simulink model "DYC_autosar"  (R2019b)
settings: Solver=VariableStepAuto  StartTime=0.0  StopTime=10.0  RelTol=1e-3
values from neighbouring files (symbols this model uses):
  Caf = 460.0    [VehCtrlMdelDictionary.sldd]
  Car = 440.0    [VehCtrlMdelDictionary.sldd]
  dwf = 1.2    [VehCtrlMdelDictionary.sldd]
  Iz = 105.0    [VehCtrlMdelDictionary.sldd]
  Ki = 1.0    [VehCtrlMdelDictionary.sldd]
  Kp = 2.0    [VehCtrlMdelDictionary.sldd]
  lf = 0.761    [VehCtrlMdelDictionary.sldd]
  lr = 0.831    [VehCtrlMdelDictionary.sldd]
  m = 340.0    [VehCtrlMdelDictionary.sldd]
  Rt = 0.2    [VehCtrlMdelDictionary.sldd]
libraries: simulink x4
settings Model: Creator=12045  LastModifiedBy=12045
settings OptimizationCC: DefaultParameterBehavior=Inlined  EnhancedBackFolding=on  PassReuseOutputArgsAs=Individual arguments  ZeroExternalMemoryAtStartup=off  ZeroInternalMemoryAtStartup=off  OptimizeBlockOrder=speed  DifferentSizesBufferReuse=on  OptimizationCustomize=off  EfficientTunableParamExpr=on
settings DebuggingCC: ParameterTunabilityLossMsg=error
settings SFSimCC: MATLABDynamicMemAlloc=off
settings RTWCC: Description=AUTOSAR  SystemTargetFile=autosar.tlc  GenCodeOnly=on  TemplateMakefile=ert_default_tmf  GenerateReport=on  IncludeHyperlinkInReport=on  LaunchReport=on  GenerateTraceInfo=on  GenerateTraceReport=on  GenerateTraceReportSl=on  GenerateTraceReportSf=on  GenerateTraceReportEml=on
settings CodeAppCC: ForceParamTrailComments=on  IgnoreCustomStorageClasses=off  OperatorAnnotations=on  SimulinkDataObjDesc=on  SFDataObjDesc=on  InsertBlockDesc=on
settings STFCustomTargetCC: TargetLangStandard=C99 (ISO)  MultiwordLength=256  ParMdlRefBuildCompliant=on  CompOptLevelCompliant=on  IncludeMdlTerminateFcn=off  CombineOutputUpdateFcns=on  SuppressErrorStatus=on  ERTCustomFileBanners=on  SupportNonFinite=off  SupportComplex=off  SupportContinuousTime=off  SupportNonInlinedSFcns=off  RemoveResetFunc=on  MATLABClassNameForMDSCustomization=Simulink.SoftwareTarget.ERTCustomization  AutosarCompliant=on  UseToolchainInfoCompliant=on  LookupTableObjectStructAxisOrder=2,1,3,4,...  LUTObjectStructOrderEvenSpacing=Size,Table,Breakpoints  SystemTargetFile=autosar.tlc
settings ERTTargetCC: TargetLangStandard=C99 (ISO)  ConcurrentExecutionCompliant=off  IncludeMdlTerminateFcn=off  SuppressErrorStatus=on  SupportNonFinite=off  SupportComplex=off  ModelStepFunctionPrototypeControlCompliant=off  CPPClassGenCompliant=off  AutosarCompliant=on  LookupTableObjectStructAxisOrder=2,1,3,4,...  LUTObjectStructOrderEvenSpacing=Size,Table,Breakpoints  InlinedParameterPlacement=NonHierarchical  ERTCustomFileTemplate=example_file_process.tlc

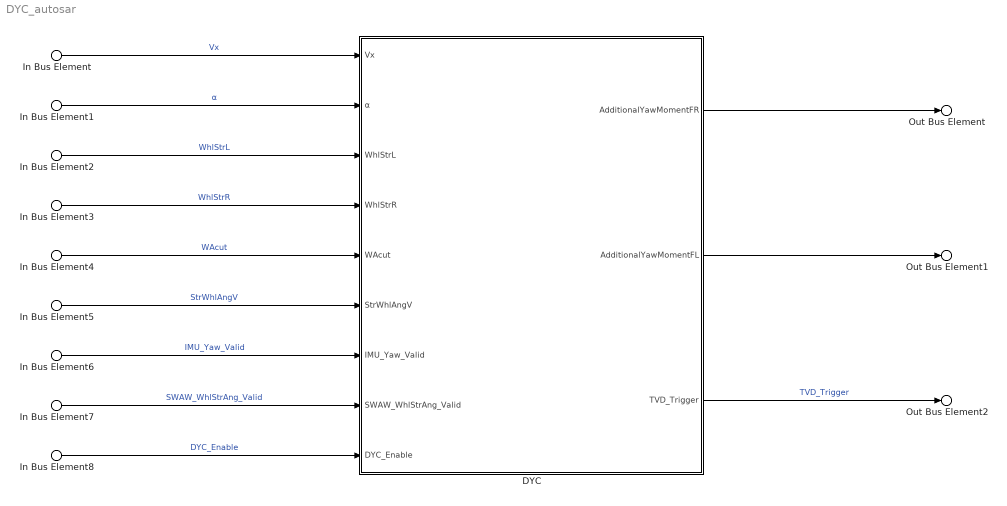
== system DYC_autosar ==
  In Bus Element : Inport  PortName=Vx  Element=Vx
  In Bus Element1 : Inport  Port=2  PortName=x0x03B1  Element=x0x03B1
  In Bus Element2 : Inport  Port=3  PortName=WhlStrL  Element=WhlStrL
  In Bus Element3 : Inport  Port=4  PortName=WhlStrR  Element=WhlStrR
  In Bus Element4 : Inport  Port=5  PortName=WAcut  Element=WAcut
  In Bus Element5 : Inport  Port=6  PortName=StrWhlAngV  Element=StrWhlAngV
  In Bus Element6 : Inport  Port=7  PortName=IMU_Yaw_Valid  Element=IMU_Yaw_Valid
  In Bus Element7 : Inport  Port=8  PortName=SWAW_WhlStrAng_Valid  Element=SWAW_WhlStrAng_Valid
  In Bus Element8 : Inport  Port=9  PortName=DYC_Enable  Element=DYC_Enable
  DYC : Subsystem
  Out Bus Element : Outport  PortName=TrqR_cmd  Element=TrqR_cmd
  Out Bus Element1 : Outport  Port=2  PortName=TrqR_cmd1  Element=TrqR_cmd1
  Out Bus Element2 : Outport  Port=3  PortName=TVD_Trigger  Element=TVD_Trigger
  wires:
  In Bus Element/1 -> DYC/1(Vx)  "Vx"
  In Bus Element1/1 -> DYC/2(α)  "α"
  In Bus Element2/1 -> DYC/3(WhlStrL)  "WhlStrL"
  In Bus Element3/1 -> DYC/4(WhlStrR)  "WhlStrR"
  In Bus Element4/1 -> DYC/5(WAcut)  "WAcut"
  In Bus Element5/1 -> DYC/6(StrWhlAngV)  "StrWhlAngV"
  In Bus Element6/1 -> DYC/7(IMU_Yaw_Valid)  "IMU_Yaw_Valid"
  In Bus Element7/1 -> DYC/8(SWAW_WhlStrAng_Valid)  "SWAW_WhlStrAng_Valid"
  In Bus Element8/1 -> DYC/9("DYC_Enable ")  "DYC_Enable"
  DYC/1(AdditionalYawMomentFR) -> Out Bus Element/1
  DYC/2(AdditionalYawMomentFL) -> Out Bus Element1/1
  DYC/3(TVD_Trigger) -> Out Bus Element2/1  "TVD_Trigger"

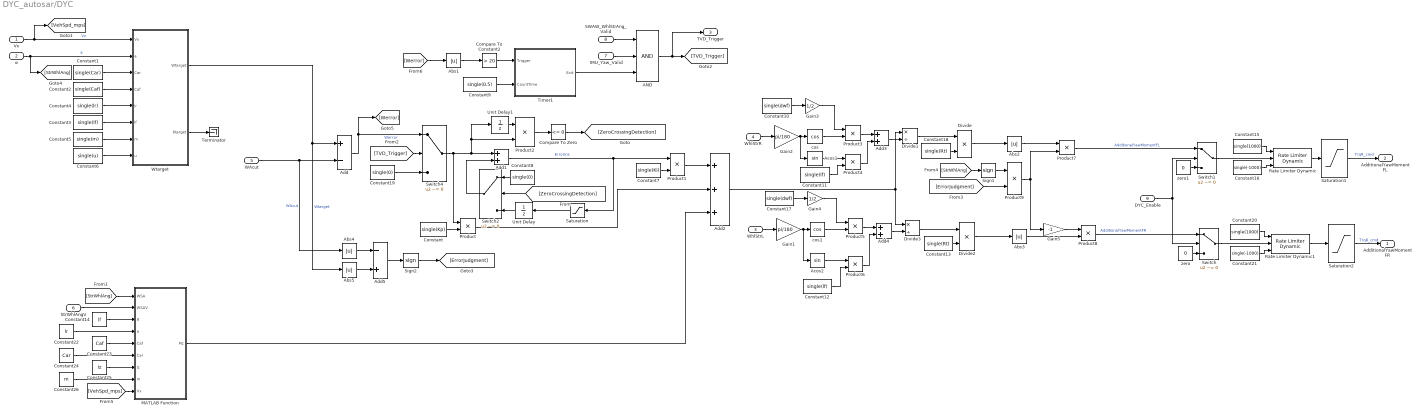
== system DYC_autosar/DYC ==
  Vx : Inport
  α : Inport  Port=2
  WhlStrL : Inport  Port=3
  WhlStrR : Inport  Port=4
  WAcut : Inport  Port=5
  StrWhlAngV : Inport  Port=6
  IMU_Yaw_Valid : Inport  Port=7
  SWAW_WhlStrAng_Valid : Inport  Port=8
  "DYC_Enable " : Inport  Port=9
  AND : Logic  Inputs=3  AllPortsSameDT=off  OutDataTypeStr=boolean
  Abs{1..5} (5 alike) : Abs
  Acos1 : Trigonometry
  Acos2 : Trigonometry
  Add : Sum  Inputs=+-
  Add1 : Sum
  Add2 : Sum  Inputs=+++
  Add3 : Sum
  Add4 : Sum
  Add5 : Sum  Inputs=-+
  Compare To Constant2 : simulink/Logic and Bit Operations/Compare To Constant  relop=>  const=20  OutDataTypeStr=boolean
  Compare To Zero : simulink/Logic and Bit Operations/Compare To Zero  relop=<=  OutDataTypeStr=boolean
  Constant : Constant  Value=single(Kp)
  Constant1 : Constant  Value=single(Car)
  Constant10 : Constant  Value=single(dwf)
  Constant11 : Constant  Value=single(lf)
  Constant12 : Constant  Value=single(lf)
  Constant13 : Constant  Value=single(Rt)
  Constant14 : Constant  Value=lf
  Constant15 : Constant  Value=single(1000)
  Constant16 : Constant  Value=single(-1000)
  Constant17 : Constant  Value=single(dwf)
  Constant18 : Constant  Value=single(Rt)
  Constant19 : Constant  Value=single(0)
  Constant2 : Constant  Value=single(Caf)
  Constant20 : Constant  Value=single(1000)
  Constant21 : Constant  Value=single(-1000)
  Constant22 : Constant  Value=lr
  Constant23 : Constant  Value=Caf
  Constant24 : Constant  Value=Car
  Constant25 : Constant  Value=Iz
  Constant26 : Constant  Value=m
  Constant3 : Constant  Value=single(lf)
  Constant4 : Constant  Value=single(lr)
  Constant5 : Constant  Value=single(m)
  Constant6 : Constant  Value=single(u)
  Constant7 : Constant  Value=single(Ki)
  Constant8 : Constant  Value=single(0)
  Constant9 : Constant  Value=single(0.5)
  Divide : Product  Inputs=**
  Divide1 : Product  Inputs=*/
  Divide2 : Product  Inputs=**
  Divide3 : Product  Inputs=*/
  Gain1 : Gain  Gain=pi/180
  Gain2 : Gain  Gain=pi/180
  Gain3 : Gain  Gain=1/2
  Gain4 : Gain  Gain=1/2
  Gain5 : Gain  Gain=-1
  MATLAB Function : MATLAB Function  TreatAsAtomicUnit=on
  Product{,1..9} (10 alike) : Product
  Rate Limiter Dynamic : simulink/Discontinuities/Rate Limiter Dynamic
      settings: SourceProductName=Simulink
  Rate Limiter Dynamic1 : simulink/Discontinuities/Rate Limiter Dynamic
      settings: SourceProductName=Simulink
  Saturation : Saturate  UpperLimit=10  LowerLimit=-10
  Saturation1 : Saturate  UpperLimit=20  LowerLimit=-20
  Saturation2 : Saturate  UpperLimit=20  LowerLimit=-20
  Sign1 : Signum
  Sign2 : Signum
  Switch{,1..2,4} (4 alike) : Switch  Criteria=u2 ~= 0
  Terminator : Terminator
  Timer1 : Stateflow chart  TreatAsAtomicUnit=on
  Unit Delay : UnitDelay  SampleTime=-1  HasFrameUpgradeWarning=on
  Unit Delay1 : UnitDelay  SampleTime=-1  HasFrameUpgradeWarning=on
  Wtarget : MATLAB Function  TreatAsAtomicUnit=on
  cos : Trigonometry  Operator=cos
  cos1 : Trigonometry  Operator=cos
  zero : Constant  Value=0
  zero1 : Constant  Value=0
  AdditionalYawMomentFR : Outport  VectorParamsAs1DForOutWhenUnconnected=off
  AdditionalYawMomentFL : Outport  Port=2  VectorParamsAs1DForOutWhenUnconnected=off
  TVD_Trigger : Outport  Port=3  VectorParamsAs1DForOutWhenUnconnected=off
  wires:
  Constant2/1 -> Wtarget/4(Caf)
  Wtarget/1(Wtarget) -> Add/1, Abs5/1  "Wtarget"
  Vx/1 -> [VehSpd_mps], Wtarget/1(Vx)  "Vx"
  Constant6/1 -> Wtarget/8(u)
  Constant5/1 -> Wtarget/7(m)
  Constant1/1 -> Wtarget/3(Car)
  Constant3/1 -> Wtarget/6(lf)
  α/1 -> [StrWhlAng], Wtarget/2(a)  "a"
  Constant4/1 -> Wtarget/5(lr)
  Product8/1 -> Switch/1  "AdditionalYawMomentFR"
  Product7/1 -> Switch1/1  "AdditionalYawMomentFL"
  Wtarget/2(btarget) -> Terminator/1
  Switch/1 -> Rate Limiter Dynamic1/2
  Switch1/1 -> Rate Limiter Dynamic/2
  "DYC_Enable "/1 -> Switch1/2, Switch/2
  zero/1 -> Switch/3
  zero1/1 -> Switch1/3
  Compare To Zero/1 -> [ZeroCrossingDetection]
  Abs3/1 -> Product8/2
  Abs5/1 -> Add5/2
  Abs4/1 -> Add5/1
  Constant19/1 -> Switch4/3
  Add5/1 -> Sign2/1
  Constant12/1 -> Product6/2
  Sign2/1 -> [ErrorJudgment]
  Saturation/1 -> Unit Delay/1
  Divide/1 -> Abs2/1
  [ErrorJudgment] -> Product9/2
  Unit Delay/1 -> Switch2/3
  Add1/1 -> Saturation/1, Product1/1  "ErrorIns"
  Add3/1 -> Divide1/2
  Gain5/1 -> Product8/1
  Product4/1 -> Add3/2
  Abs2/1 -> Product7/1
  Acos2/1 -> Product6/1
  Add/1 -> [Werror], Switch4/1  "Werror"
  Gain1/1 -> cos1/1, Acos2/1
  Constant15/1 -> Rate Limiter Dynamic/1
  Divide1/1 -> Divide/1
  WhlStrL/1 -> Gain1/1
  cos/1 -> Product3/2
  [TVD_Trigger] -> Switch4/2
  Constant11/1 -> Product4/2
  Product5/1 -> Add4/1
  Product3/1 -> Add3/1
  Constant10/1 -> Gain3/1
  Gain2/1 -> Acos1/1, cos/1
  Gain3/1 -> Product3/1
  Constant8/1 -> Switch2/1
  Product6/1 -> Add4/2
  Acos1/1 -> Product4/1
  WhlStrR/1 -> Gain2/1
  Add4/1 -> Divide3/2
  Constant18/1 -> Divide/2
  Constant17/1 -> Gain4/1
  Switch4/1 -> Add1/1, Unit Delay1/1, Product2/2, Product/1
  WAcut/1 -> Add/2, Abs4/1  "WAcut"
  Product/1 -> Add2/2
  Abs1/1 -> Compare To Constant2/1
  [ZeroCrossingDetection] -> Switch2/2
  Compare To Constant2/1 -> Timer1/1(Trigger)
  Divide3/1 -> Divide2/1
  Gain4/1 -> Product5/1
  Constant13/1 -> Divide2/2
  Switch2/1 -> Add1/2
  Product9/1 -> Gain5/1, Product7/2
  cos1/1 -> Product5/2
  Constant16/1 -> Rate Limiter Dynamic/3
  Sign1/1 -> Product9/1
  Divide2/1 -> Abs3/1
  Constant/1 -> Product/2
  Constant7/1 -> Product1/2
  Product1/1 -> Add2/1
  Rate Limiter Dynamic/1 -> Saturation1/1
  Constant21/1 -> Rate Limiter Dynamic1/3
  Constant20/1 -> Rate Limiter Dynamic1/1
  Rate Limiter Dynamic1/1 -> Saturation2/1
  Add2/1 -> Divide3/1, Divide1/1
  Saturation1/1 -> AdditionalYawMomentFL/1  "TrqR_cmd"
  Saturation2/1 -> AdditionalYawMomentFR/1  "TrqR_cmd"
  [StrWhlAng] -> Sign1/1
  StrWhlAngV/1 -> MATLAB Function/2(WSAV)
  Constant9/1 -> Timer1/2(CountTime)
  Timer1/1(Exit) -> AND/3
  IMU_Yaw_Valid/1 -> AND/2
  SWAW_WhlStrAng_Valid/1 -> AND/1
  AND/1 -> TVD_Trigger/1, [TVD_Trigger]
  MATLAB Function/1(Mz) -> Add2/3
  [StrWhlAng] -> MATLAB Function/1(WSA)
  Constant14/1 -> MATLAB Function/3(lf)
  Constant22/1 -> MATLAB Function/4(lr)
  Constant23/1 -> MATLAB Function/5(Caf)
  Constant24/1 -> MATLAB Function/6(Car)
  Constant25/1 -> MATLAB Function/7(Iz)
  Constant26/1 -> MATLAB Function/8(m)
  [VehSpd_mps] -> MATLAB Function/9(Vx)
  Unit Delay1/1 -> Product2/1
  Product2/1 -> Compare To Zero/1
  [Werror] -> Abs1/1

== matlab function DYC_autosar/DYC/Wtarget ==
  data: Vx input size=1; Wtarget output size=1; a input size=1; Car input size=1; Caf input size=1; lr input size=1; lf input size=1; m input; u input; btarget output
function [Wtarget,btarget] = fcn(Vx,a,Car,Caf,lr,lf,m,u)
Wdes = Vx*a/(lf+lr+(m*Vx*Vx*(lr*Car-lf*Caf)/Caf/Car/(lr+lf)/2));
% Wu = 0.85*u*9.8/Vx;
% if abs(Wdes)<=Wu
Wtarget = Wdes;
% else
%    Wtarget = Wu*sign(Wdes);
% end
bdes = (lr-lf*m*Vx*Vx/Car/(lf+lr)/2)*a/(lr+lf+m*Vx*Vx*(lr*Car-lf*Caf)/Car/Caf/(lf+lr)/2);
bu = atan(0.02*u*9.8);
if abs(bdes)<=bu
btarget = bdes;
else
    btarget = bu*sign(bdes);
end

== stateflow chart DYC_autosar/DYC/Timer1 ==
  state Trigger
    en:
    x = x + 0.01;
    Exit=0;
  state Out
    en:
    Exit=1;
    x=0;
  state InterState
    en:
    x=0;
  Trigger -> Trigger [order 1] : [Trigger&&x<CountTime]
  Trigger -> Out [order 2] : [x>=CountTime]
  (default) -> Trigger
  Out -> Trigger : [~Trigger]
  InterState -> Trigger : [Trigger]
  Trigger -> InterState [order 3] : [x<CountTime&&~Trigger]
  data: Trigger input; CountTime input; Exit output; x local =0

== matlab function DYC_autosar/DYC/MATLAB Function ==
  data: WSA input; Mz output; WSAV input; lf input; lr input; Caf input; Car input; Iz input; m input; Vx input
function Mz = fcn(WSA,WSAV,lf,lr,Caf,Car,Iz,m,Vx)

Mz = (((lf*lf*Caf+lr*lr*Car)/Iz/Vx)*(-Caf/m/Vx)-((lf*Caf-lr*Car)/m/Vx/Vx-1)*(-lf*Caf/Iz))*Iz*WSA/((lf*Caf-lr*Car)/m/Vx/Vx-1)-(-Caf/m/Vx)*Iz*WSAV/((lf*Caf-lr*Car)/m/Vx/Vx-1);
